simulink library "Compressor_StaticSimulink"  (R2013b)
settings: Solver=ode45  StartTime=0.0  StopTime=10.0  RelTol=1e-3
libraries: Compressor_StaticSimulink x4, simulink x1
settings Model: Creator=mbrauer  LastModifiedBy=mbrauer

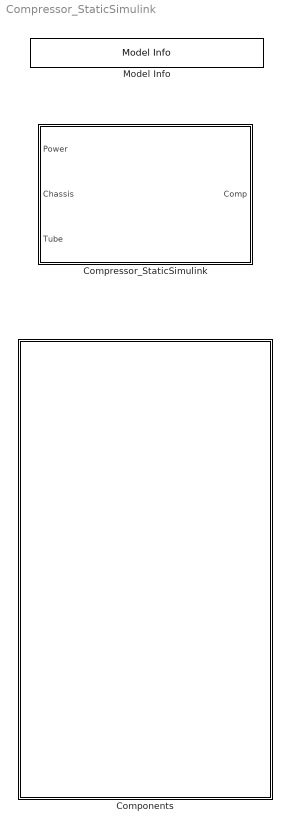
== system Compressor_StaticSimulink ==
  Components : Subsystem
  Compressor_StaticSimulink : Subsystem
  Model Info : simulink/Model-Wide Utilities/Model Info  InitialBlockCM=None  BlockCM=None  Frame=on  DisplayStringWithTags=Copyright 2013-2014 The MathWorks, Inc.  HorizontalTextAlignment=Center  LeftAlignmentValue=0.5  SourceBlockDiagram=Compressor_StaticSimulink  TagMaxNumber=20

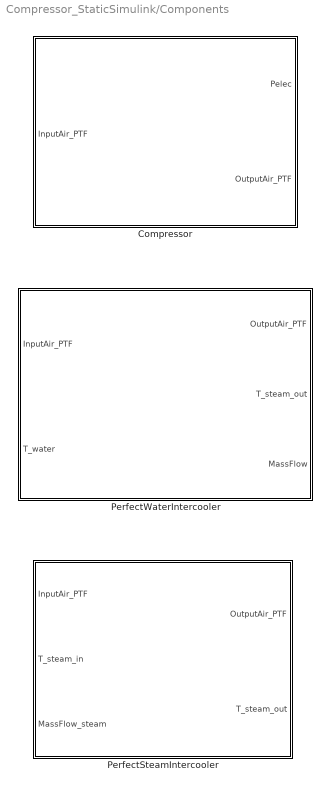
== system Compressor_StaticSimulink/Components ==
  Compressor : Subsystem  mask(Compressor){CPR=21, nc=0.75}
      mask prompts: CPR "Compression Ratio"; nc "Efficiency"
      mask help:
      | Basic compressor model, including electric motor.
      |
      | Determines output air pressure and temperature based on defined Compression ratio. Also determines required electrical power.
      mask init:
      | if or(nc > 1,nc<=0)
      |     error('nc should be a value between 0 and 1')
      | end
      | 
      | cp_air = 1e3; 
      | gamma = 1.4;
      mask Display: image('CompressorIcon.png',[80 30 110 140])
  PerfectSteamIntercooler : Subsystem  mask(Intercooler){T_air_out=400, eff=0.6}
      mask prompts: T_air_out "Target Output Temperature"; eff "Efficiency"
      mask help:
      | Basic intercooler model, for air to water heat exchange
      |
      | Calculates power to cool input air to desired temperature and converts that heat to water/steam.
      mask init:
      | cp_air      = 1e3;     % J/kg/K
      | cp_steam    = 1.996e3; % J/kg/K
      | T_steam     = 373;
      | if or(eff > 1,eff<=0)
      |     error('eff should be a value between 0 and 1')
      | end
      mask Display: image('Intercooler.png',[70 20 120 160])
  PerfectWaterIntercooler : Subsystem  mask(Intercooler){T_air_out=300, eff=0.6}
      mask prompts: T_air_out "Target Output Temperature"; eff "Efficiency"
      mask help:
      | Basic intercooler model, for air to water heat exchange
      |
      | Calculates power to cool input air to desired temperature and converts that heat to water/steam.
      mask init:
      | cp_air      = 1e3;     % J/kg/K
      | cp_steam    = 1.996e3; % J/kg/K
      | cp_water    = 4.186e3; % J/kg/K
      | W_H20_L2V   = 40.7e6/18; % J/kg (40.7 kJ/mol / 18 g/mol)
      | T_steam     = 373;
      | if or(eff > 1,eff<=0)
      |     error('eff should be a value between 0 and 1')
      | end
      mask Display: image('Intercooler.png',[60 10 170 180])

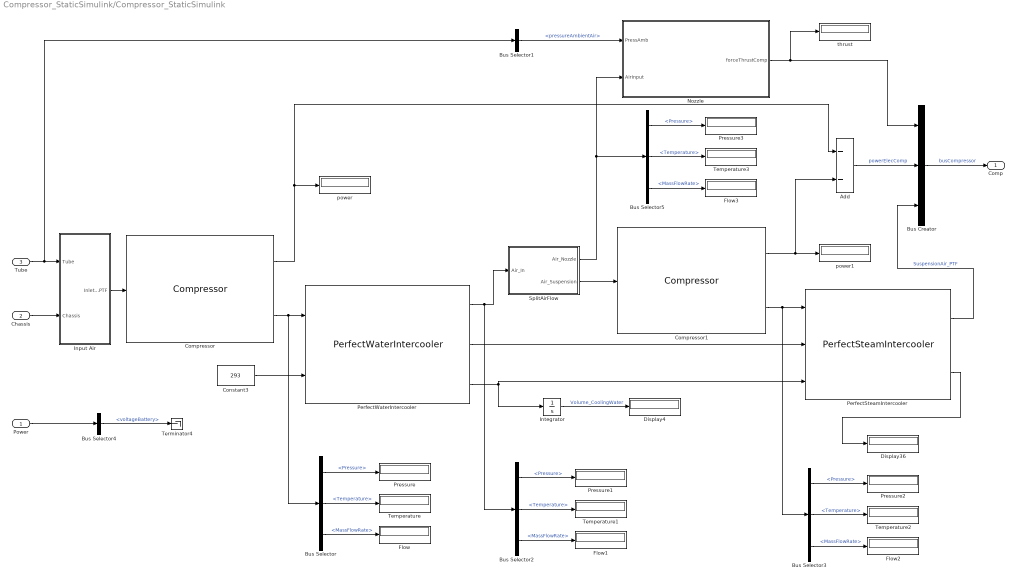
== system Compressor_StaticSimulink/Compressor_StaticSimulink ==
  Power : Inport
  Chassis : Inport  Port=2
  Tube : Inport  Port=3
  Add : Sum  Inputs=--
  Bus Creator : BusCreator  Inputs=3  NonVirtualBus=on
  Bus Selector{,2..3,5} (4 alike) : BusSelector  OutputSignals=Pressure,Temperature,MassFlowRate
  Bus Selector1 : BusSelector  OutputSignals=pressureAmbientAir
  Bus Selector4 : BusSelector  OutputSignals=voltageBattery
  Compressor : Compressor_StaticSimulink/Components/Compressor  CPR=21  nc=0.75
  Compressor1 : Compressor_StaticSimulink/Components/Compressor  CPR=21  nc=0.75
  Constant3 : Constant  Value=293
  Display36 : Display
  Display4 : Display
  Flow{,1..3} (4 alike) : Display
      settings: Decimation=100
  Input Air : Subsystem
  Integrator : Integrator
  Nozzle : Subsystem
  PerfectSteamIntercooler : Compressor_StaticSimulink/Components/PerfectSteamIntercooler  T_air_out=400  eff=0.6
  PerfectWaterIntercooler : Compressor_StaticSimulink/Components/PerfectWaterIntercooler  T_air_out=300  eff=0.6
  Pressure{,1..3} (4 alike) : Display
      settings: Decimation=100
  SplitAirFlow : Subsystem
  Temperature{,1..3} (4 alike) : Display
      settings: Decimation=100
  Terminator4 : Terminator
  power : Display
  power1 : Display
  thrust : Display
  Comp : Outport
  wires:
  Bus Selector5/3 -> Flow3/1  "<MassFlowRate>"
  Bus Selector5/1 -> Pressure3/1  "<Pressure>"
  Bus Selector5/2 -> Temperature3/1  "<Temperature>"
  Bus Selector3/3 -> Flow2/1  "<MassFlowRate>"
  Bus Selector3/1 -> Pressure2/1  "<Pressure>"
  Bus Selector3/2 -> Temperature2/1  "<Temperature>"
  Bus Selector2/3 -> Flow1/1  "<MassFlowRate>"
  Bus Selector2/1 -> Pressure1/1  "<Pressure>"
  Bus Selector2/2 -> Temperature1/1  "<Temperature>"
  Bus Selector/3 -> Flow/1  "<MassFlowRate>"
  Bus Selector/1 -> Pressure/1  "<Pressure>"
  Bus Selector/2 -> Temperature/1  "<Temperature>"
  PerfectSteamIntercooler/1 -> Bus Creator/3  "SuspensionAir_PTF"
  Compressor1/2 -> PerfectSteamIntercooler/1, Bus Selector3/1
  Input Air/1(InletAir_PTF) -> Compressor/1
  Bus Selector1/1 -> Nozzle/1(PressAmb)  "<pressureAmbientAir>"
  SplitAirFlow/1(Air_Nozzle) -> Bus Selector5/1, Nozzle/2(AirInput)
  PerfectWaterIntercooler/1 -> Bus Selector2/1, SplitAirFlow/1(Air_In)
  Compressor/1 -> Add/1, power/1
  Compressor1/1 -> Add/2, power1/1
  PerfectSteamIntercooler/2 -> Display36/1
  Integrator/1 -> Display4/1  "Volume_CoolingWater"
  PerfectWaterIntercooler/3 -> PerfectSteamIntercooler/3, Integrator/1
  PerfectWaterIntercooler/2 -> PerfectSteamIntercooler/2
  SplitAirFlow/2(Air_Suspension) -> Compressor1/1
  Compressor/2 -> PerfectWaterIntercooler/1, Bus Selector/1
  Constant3/1 -> PerfectWaterIntercooler/2
  Bus Selector4/1 -> Terminator4/1  "<voltageBattery>"
  Power/1 -> Bus Selector4/1
  Add/1 -> Bus Creator/2  "powerElecComp"
  Bus Creator/1 -> Comp/1  "busCompressor"
  Nozzle/1(forceThrustComp) -> thrust/1, Bus Creator/1
  Tube/1 -> Bus Selector1/1, Input Air/1(Tube)
  Chassis/1 -> Input Air/2(Chassis)

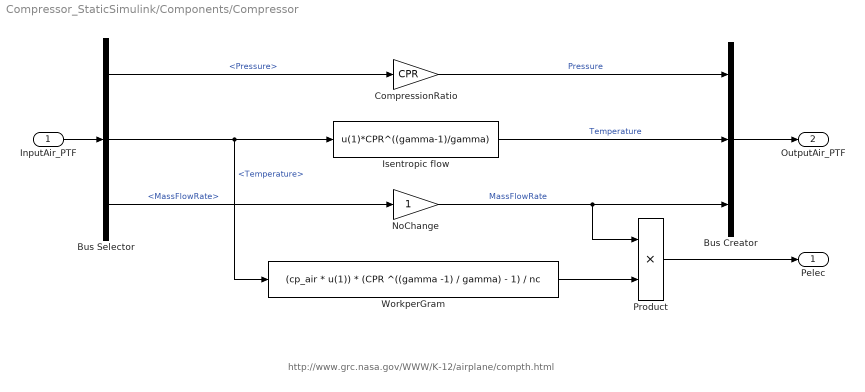
== system Compressor_StaticSimulink/Components/Compressor ==
  note: http://www.grc.nasa.gov/WWW/K-12/airplane/compth.html
  InputAir_PTF : Inport
  Bus Creator : BusCreator  Inputs=3
  Bus Selector : BusSelector  OutputSignals=Pressure,Temperature,MassFlowRate
  CompressionRatio : Gain  Gain=CPR
  Isentropic flow : Fcn  Expr=u(1)*CPR^((gamma-1)/gamma)
  NoChange : Gain
  Product : Product
  WorkperGram : Fcn  Expr=(cp_air * u(1)) * (CPR ^((gamma -1) / gamma) - 1) / nc
  Pelec : Outport
  OutputAir_PTF : Outport  Port=2
  wires:
  Isentropic flow/1 -> Bus Creator/2  "Temperature"
  Bus Selector/2 -> WorkperGram/1, Isentropic flow/1  "<Temperature>"
  Bus Selector/1 -> CompressionRatio/1  "<Pressure>"
  CompressionRatio/1 -> Bus Creator/1  "Pressure"
  WorkperGram/1 -> Product/2
  Product/1 -> Pelec/1
  NoChange/1 -> Product/1, Bus Creator/3  "MassFlowRate"
  Bus Creator/1 -> OutputAir_PTF/1
  InputAir_PTF/1 -> Bus Selector/1
  Bus Selector/3 -> NoChange/1  "<MassFlowRate>"

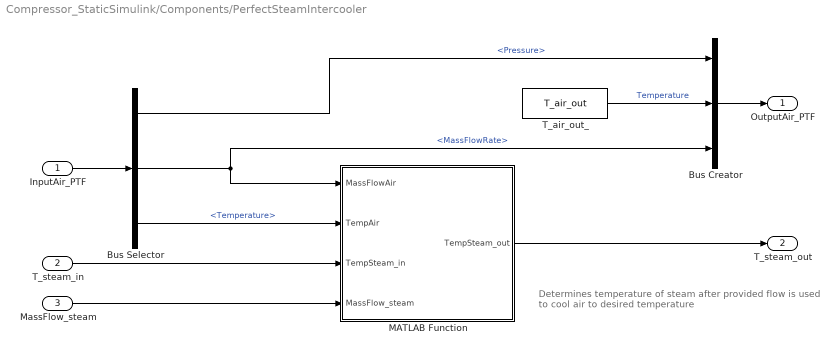
== system Compressor_StaticSimulink/Components/PerfectSteamIntercooler ==
  note: Determines temperature of steam after provided flow is
      | used to cool air to desired temperature
  InputAir_PTF : Inport
  T_steam_in : Inport  Port=2
  MassFlow_steam : Inport  Port=3
  Bus Creator : BusCreator  Inputs=3
  Bus Selector : BusSelector  OutputSignals=Pressure,MassFlowRate,Temperature
  MATLAB Function : MATLAB Function  TreatAsAtomicUnit=on
  T_air_out_ : Constant  Value=T_air_out
  OutputAir_PTF : Outport
  T_steam_out : Outport  Port=2
  wires:
  Bus Selector/3 -> MATLAB Function/2(TempAir)  "<Temperature>"
  Bus Selector/2 -> Bus Creator/3, MATLAB Function/1(MassFlowAir)  "<MassFlowRate>"
  T_air_out_/1 -> Bus Creator/2  "Temperature"
  T_steam_in/1 -> MATLAB Function/3(TempSteam_in)
  Bus Selector/1 -> Bus Creator/1  "<Pressure>"
  MassFlow_steam/1 -> MATLAB Function/4(MassFlow_steam)
  MATLAB Function/1(TempSteam_out) -> T_steam_out/1
  InputAir_PTF/1 -> Bus Selector/1
  Bus Creator/1 -> OutputAir_PTF/1

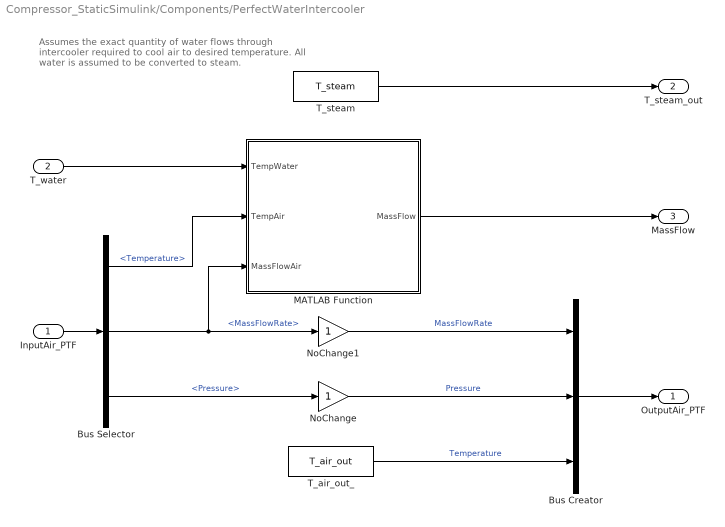
== system Compressor_StaticSimulink/Components/PerfectWaterIntercooler ==
  note: Assumes the exact quantity of water flows through
      | intercooler required to cool air to desired temperature.
      | All water is assumed to be converted to steam.
  InputAir_PTF : Inport
  T_water : Inport  Port=2
  Bus Creator : BusCreator  Inputs=3
  Bus Selector : BusSelector  OutputSignals=Temperature,MassFlowRate,Pressure
  MATLAB Function : MATLAB Function  TreatAsAtomicUnit=on
  NoChange : Gain
  NoChange1 : Gain
  T_air_out_ : Constant  Value=T_air_out
  T_steam : Constant  Value=T_steam
  OutputAir_PTF : Outport
  T_steam_out : Outport  Port=2
  MassFlow : Outport  Port=3
  wires:
  T_steam/1 -> T_steam_out/1
  MATLAB Function/1(MassFlow) -> MassFlow/1
  T_water/1 -> MATLAB Function/1(TempWater)
  InputAir_PTF/1 -> Bus Selector/1
  Bus Selector/3 -> NoChange/1  "<Pressure>"
  Bus Selector/1 -> MATLAB Function/2(TempAir)  "<Temperature>"
  Bus Selector/2 -> MATLAB Function/3(MassFlowAir), NoChange1/1  "<MassFlowRate>"
  T_air_out_/1 -> Bus Creator/3  "Temperature"
  NoChange/1 -> Bus Creator/2  "Pressure"
  NoChange1/1 -> Bus Creator/1  "MassFlowRate"
  Bus Creator/1 -> OutputAir_PTF/1

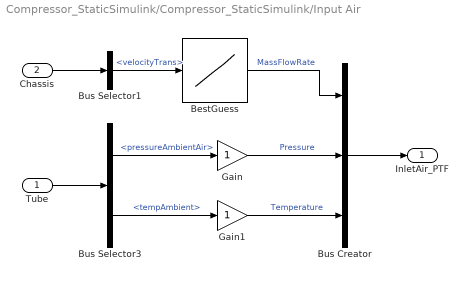
== system Compressor_StaticSimulink/Compressor_StaticSimulink/Input Air ==
  Tube : Inport
  Chassis : Inport  Port=2
  BestGuess : Lookup_n-D  NumberOfTableDimensions=1  BreakpointsForDimension1=[0 100 340 400]  Table=[0.3 0.3 0.49 0.49]  ExtrapMethod=Clip  UseLastTableValue=on  InternalRulePriority=Speed  RndMeth=Simplest  InputSameDT=on
  Bus Creator : BusCreator  Inputs=3
  Bus Selector1 : BusSelector  OutputSignals=velocityTrans
  Bus Selector3 : BusSelector  OutputSignals=pressureAmbientAir,tempAmbient
  Gain : Gain
  Gain1 : Gain
  InletAir_PTF : Outport
  wires:
  Tube/1 -> Bus Selector3/1
  Bus Selector3/1 -> Gain/1  "<pressureAmbientAir>"
  Bus Selector3/2 -> Gain1/1  "<tempAmbient>"
  BestGuess/1 -> Bus Creator/1  "MassFlowRate"
  Chassis/1 -> Bus Selector1/1
  Bus Selector1/1 -> BestGuess/1  "<velocityTrans>"
  Gain/1 -> Bus Creator/2  "Pressure"
  Bus Creator/1 -> InletAir_PTF/1
  Gain1/1 -> Bus Creator/3  "Temperature"

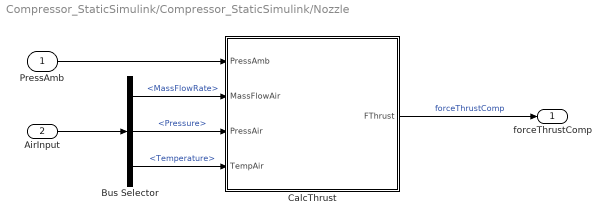
== system Compressor_StaticSimulink/Compressor_StaticSimulink/Nozzle ==
  PressAmb : Inport
  AirInput : Inport  Port=2
  Bus Selector : BusSelector  OutputSignals=MassFlowRate,Pressure,Temperature
  CalcThrust : MATLAB Function  TreatAsAtomicUnit=on
  forceThrustComp : Outport
  wires:
  Bus Selector/1 -> CalcThrust/2(MassFlowAir)  "<MassFlowRate>"
  PressAmb/1 -> CalcThrust/1(PressAmb)
  Bus Selector/3 -> CalcThrust/4(TempAir)  "<Temperature>"
  Bus Selector/2 -> CalcThrust/3(PressAir)  "<Pressure>"
  CalcThrust/1(FThrust) -> forceThrustComp/1  "forceThrustComp"
  AirInput/1 -> Bus Selector/1

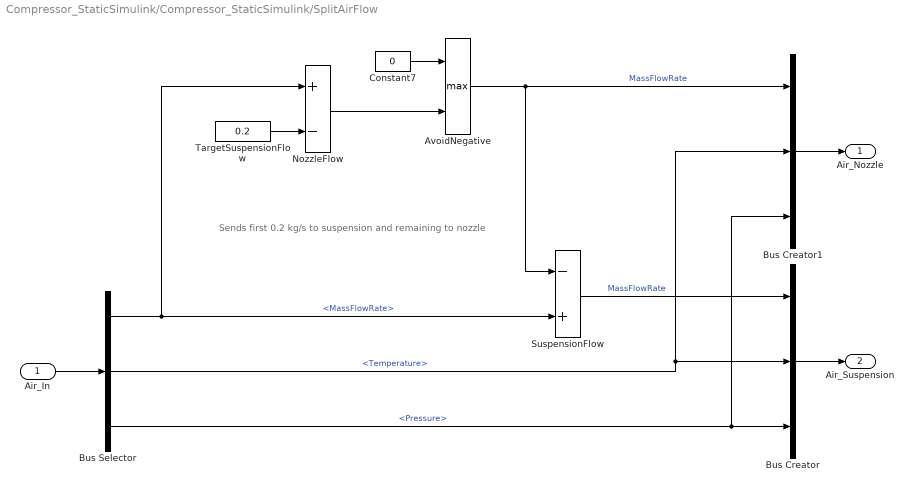
== system Compressor_StaticSimulink/Compressor_StaticSimulink/SplitAirFlow ==
  note: Sends first 0.2 kg/s to suspension and remaining to nozzle
  Air_In : Inport
  AvoidNegative : MinMax  Function=max  Inputs=2
  Bus Creator : BusCreator  Inputs=3
  Bus Creator1 : BusCreator  Inputs=3
  Bus Selector : BusSelector  OutputSignals=MassFlowRate,Temperature,Pressure
  Constant7 : Constant  Value=0
  NozzleFlow : Sum  Inputs=+-
  SuspensionFlow : Sum  Inputs=-+
  TargetSuspensionFlow : Constant  Value=0.2
  Air_Nozzle : Outport
  Air_Suspension : Outport  Port=2
  wires:
  AvoidNegative/1 -> Bus Creator1/1, SuspensionFlow/1  "MassFlowRate"
  Constant7/1 -> AvoidNegative/1
  NozzleFlow/1 -> AvoidNegative/2
  Bus Selector/1 -> NozzleFlow/1, SuspensionFlow/2  "<MassFlowRate>"
  TargetSuspensionFlow/1 -> NozzleFlow/2
  Air_In/1 -> Bus Selector/1
  Bus Creator/1 -> Air_Suspension/1
  Bus Selector/2 -> Bus Creator/2, Bus Creator1/2  "<Temperature>"
  Bus Selector/3 -> Bus Creator1/3, Bus Creator/3  "<Pressure>"
  Bus Creator1/1 -> Air_Nozzle/1
  SuspensionFlow/1 -> Bus Creator/1  "MassFlowRate"

== matlab function Compressor_StaticSimulink/Nozzle/CalcThrust ==
  data: PressAmb input; MassFlowAir input; PressAir input; TempAir input; FThrust output
function FThrust = fcn(PressAmb, MassFlowAir, PressAir, TempAir  )
%#codegen

% Parameters
gam     = 1.4;  
Rgas    = 287.04;  % J/kg/K

Ve = sqrt(2 * Rgas * gam/(gam-1) * TempAir * (1 - (PressAmb/PressAir)^((gam-1)/gam)));
% Ref http://www.braeunig.us/space/propuls.htm

FThrust = MassFlowAir*Ve;

== matlab function Compressor_StaticSimulink/Components/PerfectSteamIntercooler/MATLAB Function ==
  data: MassFlowAir input; TempSteam_out output; TempAir input; TempSteam_in input; MassFlow_steam input; cp_air parameter; T_air_out parameter; eff parameter; cp_steam parameter
function TempSteam_out = fcn(MassFlowAir,TempAir, TempSteam_in, MassFlow_steam, cp_air, T_air_out, eff, cp_steam)
%#codegen

% Heat flow to cool air to desired temperature
Qcool           = MassFlowAir*cp_air*(TempAir-T_air_out)/eff;  

TempSteam_out   = TempSteam_in + Qcool/(cp_steam*MassFlow_steam);

== matlab function Compressor_StaticSimulink/Components/PerfectWaterIntercooler/MATLAB Function ==
  data: TempWater input; TempAir input; MassFlowAir input; MassFlow output; cp_air parameter; T_air_out parameter; T_steam parameter; cp_water parameter; eff parameter; W_H20_L2V parameter
function MassFlow = fcn(TempWater,TempAir,MassFlowAir, cp_air, T_air_out, T_steam, cp_water, eff, W_H20_L2V)
%#codegen

% Mass (kg)
% Cp   (j/g/K)

% Heat flow to cool air to desired temperature
Qcool       = MassFlowAir*cp_air*(TempAir-T_air_out)/eff;  

% Temperature change from inlet water to steam (assume all water used gets
% converted to steam)
DeltaTWater = T_steam - TempWater; 

% Determine amount of water needed to generate desired thermal flow based
% on assumption above
MassFlow    = Qcool/(cp_water*DeltaTWater+W_H20_L2V);
